simulink model "Stateflow_SDfixpoint"  (R2015b)
settings: Solver=FixedStepDiscrete  StartTime=0.0  StopTime=10.0  RelTol=1e-3
settings Model: Creator=amyyang  LastModifiedBy=amyyang
settings OptimizationCC: DefaultParameterBehavior=Inlined  OptimizeModelRefInitCode=on  LifeSpan=1
settings DebuggingCC: SFUnusedDataAndEventsDiag=error
settings RTWCC: SystemTargetFile=ert.tlc  GenCodeOnly=on  TemplateMakefile=ert_default_tmf  Description=Embedded Coder  GenerateReport=on  IncludeHyperlinkInReport=on  LaunchReport=on  GenerateTraceInfo=on  GenerateTraceReport=on  GenerateTraceReportSl=on  GenerateTraceReportSf=on  GenerateTraceReportEml=on
settings CodeAppCC: IgnoreCustomStorageClasses=off
settings ERTTargetCC: GenerateSampleERTMain=on  InlinedParameterPlacement=NonHierarchical  ERTCustomFileTemplate=example_file_process.tlc

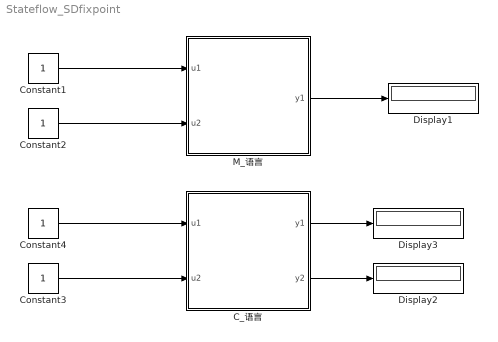
== system Stateflow_SDfixpoint ==
  C_语言 : Stateflow chart  TreatAsAtomicUnit=on
  Constant{1..4} (4 alike) : Constant  OutDataTypeStr=fixdt(1,32,30)
  Display1 : Display
  Display2 : Display
  Display3 : Display
  M_语言 : Stateflow chart  TreatAsAtomicUnit=on
  wires:
  Constant1/1 -> M_语言/1(u1)
  M_语言/1(y1) -> Display1/1
  Constant2/1 -> M_语言/2(u2)
  C_语言/2(y2) -> Display2/1
  C_语言/1(y1) -> Display3/1
  Constant4/1 -> C_语言/1(u1)
  Constant3/1 -> C_语言/2(u2)

== stateflow chart Stateflow_SDfixpoint/C_语言 ==
  (default) -> (junction 2) : {
      | %没有冒号等于
      |
      | y1 = u1 * u2;
      |
      | % 有冒号等于
      | y2 := u1 * u2;
      |
      | }
  data: y1 output double; y2 output double; u1 input; u2 input

== stateflow chart Stateflow_SDfixpoint/M_语言 ==
  (default) -> (junction 2) : {
      | %没有冒号等于
      |
      | y1 = u1 * u2;
      |
      |
      | }
  data: y1 output; u1 input; u2 input
